simulink model "model"  (R2021a)
settings: Solver=VariableStepAuto  StartTime=0.0  StopTime=T  RelTol=1e-3
values from neighbouring files (symbols this model uses):
  A = double(subs(Ap, parameters, values))    [control_d.m]
  B = double(subs(Bp, parameters, values))    [control_d.m]
  C = eye(4)    [control_d.m]
  convert_deg = diag([180/pi;180/pi;1;1])    [control_d.m]
  K = dlqr(Ad, Bd, Q, R)    [control_d.m]
  Kobs = dlqr(Ad', C', Q, R)'    [control_d.m]
  pt = cell2mat(point)'    [control_d.m]
  r = [pi/2;0;0;0]    [control_d.m]
  x0 = X0 - pt    [control_d.m]
settings Model: Creator=Usuario  LastModifiedBy=Usuario

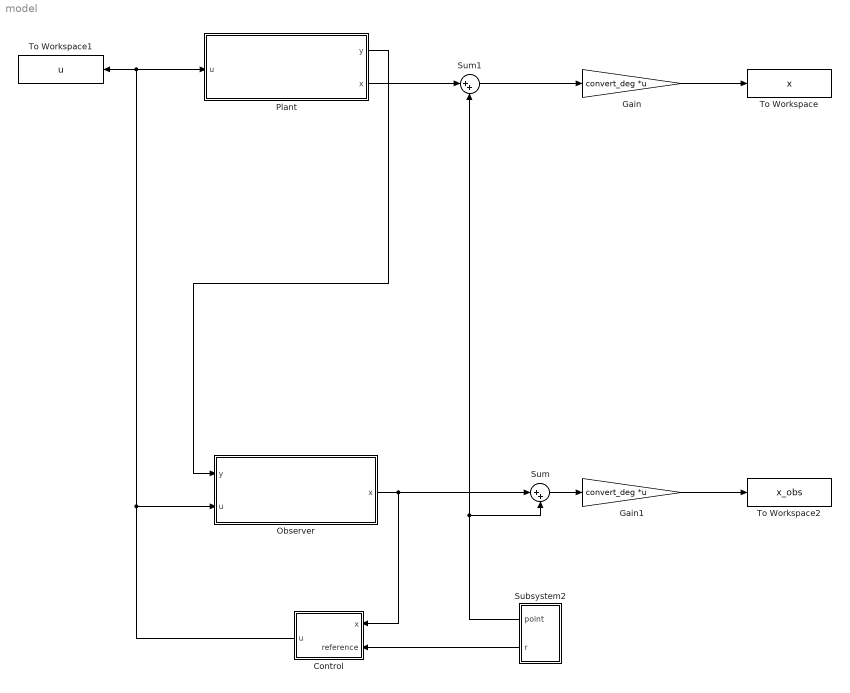
== system model ==
  Control : Subsystem
  Gain : Gain  Gain=convert_deg  Multiplication=Matrix(K*u)
  Gain1 : Gain  Gain=convert_deg  Multiplication=Matrix(K*u)
  Observer : Subsystem
  Plant : Subsystem
  Subsystem2 : Subsystem
  Sum : Sum  Inputs=|++
  Sum1 : Sum  Inputs=|++
  To Workspace : ToWorkspace  VariableName=x  SaveFormat=Timeseries  SampleTime=-1
  To Workspace1 : ToWorkspace  VariableName=u  SaveFormat=Timeseries  SampleTime=-1
  To Workspace2 : ToWorkspace  VariableName=x_obs  SaveFormat=Timeseries  SampleTime=-1
  wires:
  Plant/1(y) -> Observer/1(y)
  Plant/2(x) -> Sum1/1
  Control/1(u) -> Plant/1(u), To Workspace1/1, Observer/2(u)
  Sum1/1 -> Gain/1
  Subsystem2/1(point) -> Sum/2, Sum1/2
  Subsystem2/2(r) -> Control/2(reference)
  Gain/1 -> To Workspace/1
  Observer/1(x) -> Sum/1, Control/1(x)
  Sum/1 -> Gain1/1
  Gain1/1 -> To Workspace2/1

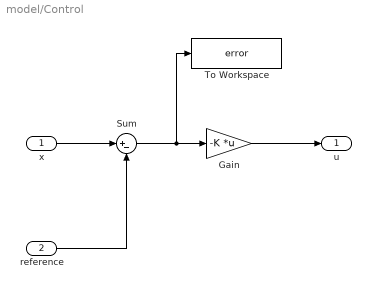
== system model/Control ==
  x : Inport
  reference : Inport  Port=2
  Gain : Gain  Gain=-K  Multiplication=Matrix(K*u)
  Sum : Sum  Inputs=|+-
  To Workspace : ToWorkspace  VariableName=error  SaveFormat=Timeseries  SampleTime=-1
  u : Outport
  wires:
  Gain/1 -> u/1
  Sum/1 -> To Workspace/1, Gain/1
  x/1 -> Sum/1
  reference/1 -> Sum/2

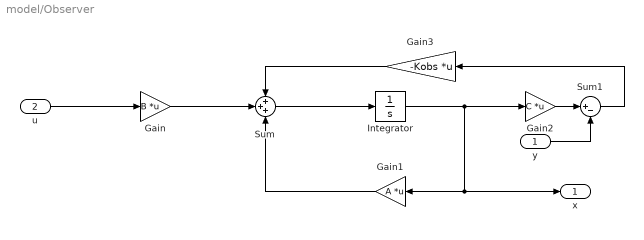
== system model/Observer ==
  y : Inport
  u : Inport  Port=2
  Gain : Gain  Gain=B  Multiplication=Matrix(K*u)
  Gain1 : Gain  Gain=A  Multiplication=Matrix(K*u)
  Gain2 : Gain  Gain=C  Multiplication=Matrix(K*u)
  Gain3 : Gain  Gain=-Kobs  Multiplication=Matrix(K*u)
  Integrator : Integrator  InitialCondition=x0
  Sum : Sum  Inputs=+++
  Sum1 : Sum  Inputs=|+-
  x : Outport
  wires:
  u/1 -> Gain/1
  Sum/1 -> Integrator/1
  Integrator/1 -> Gain1/1, x/1, Gain2/1
  Gain2/1 -> Sum1/1
  y/1 -> Sum1/2
  Sum1/1 -> Gain3/1
  Gain/1 -> Sum/2
  Gain1/1 -> Sum/3
  Gain3/1 -> Sum/1

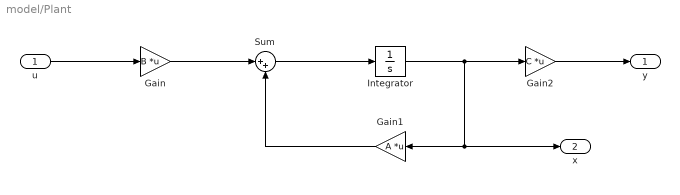
== system model/Plant ==
  u : Inport
  Gain : Gain  Gain=B  Multiplication=Matrix(K*u)
  Gain1 : Gain  Gain=A  Multiplication=Matrix(K*u)
  Gain2 : Gain  Gain=C  Multiplication=Matrix(K*u)
  Integrator : Integrator  InitialCondition=x0
  Sum : Sum  Inputs=|++
  y : Outport
  x : Outport  Port=2
  wires:
  Gain/1 -> Sum/1
  Integrator/1 -> Gain2/1, x/1, Gain1/1
  Sum/1 -> Integrator/1
  Gain1/1 -> Sum/2
  u/1 -> Gain/1
  Gain2/1 -> y/1

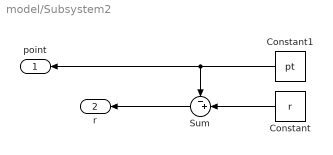
== system model/Subsystem2 ==
  Constant : Constant  Value=r
  Constant1 : Constant  Value=pt
  Sum : Sum  Inputs=-+|
  point : Outport
  r : Outport  Port=2
  wires:
  Constant1/1 -> point/1, Sum/1
  Constant/1 -> Sum/2
  Sum/1 -> r/1
